simulink model "SOC_model_Code_Gen"  (R2025a)
settings: Solver=FixedStepDiscrete  StartTime=0.0  StopTime=10.0  FixedStep=1  RelTol=1e-3
InitFcn:
  | clear
  | S = load("01_TEST_LGHG2@n10degC_Norm_(05_Inputs).mat");
  | steps = size(S.X,2);
  | t = (0:(steps-1))';
  | X_in = timeseries(single(S.X'), t);
  | true_SOC = timeseries(single(S.Y'), t);
libraries: deeplib x3
settings OptimizationCC: DefaultParameterBehavior=Inlined  EnhancedBackFolding=on  PassReuseOutputArgsAs=Individual arguments  ZeroExternalMemoryAtStartup=off  ZeroInternalMemoryAtStartup=off  OptimizeBlockOrder=speed  DifferentSizesBufferReuse=on  OptimizationCustomize=off  EfficientTunableParamExpr=on
settings DebuggingCC: ParameterTunabilityLossMsg=error
settings HardwareCC: ProdBitPerLong=64.0  ProdHWDeviceType=Intel->x86-64 (Linux 64)
settings SFSimCC: MATLABDynamicMemAlloc=off  SimTargetLang=C++  SimDLTargetLibrary=mkl-dnn
settings RTWCC: SystemTargetFile=ert.tlc  TemplateMakefile=ert_default_tmf  PortableWordSizes=on  CodeProfilingInstrumentation=coarse  Description=Embedded Coder
settings CodeAppCC: ForceParamTrailComments=on  IgnoreCustomStorageClasses=off  OperatorAnnotations=on  SimulinkDataObjDesc=on  SFDataObjDesc=on  InsertBlockDesc=on
settings ERTTargetCC: ExtModeTransport=0.0  ExtModeStaticAlloc=off  ExtModeMexFile=ext_comm  ExtModeIntrfLevel=Level1  ERTCustomFileTemplate=example_file_process.tlc  TargetLangStandard=C99 (ISO)  GenerateSampleERTMain=on  SupportVariableSizeSignals=on

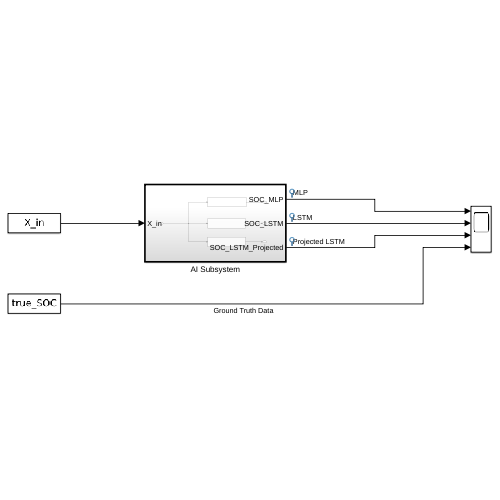
[thumbnail: Simulink's stored preview of the top-level diagram]
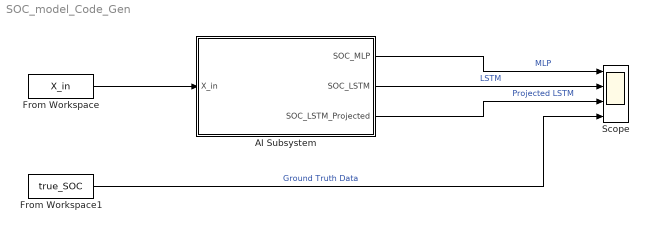
== system SOC_model_Code_Gen ==
  AI Subsystem : Subsystem  TreatAsAtomicUnit=on
      settings: RTWSystemCode=Nonreusable function
  From Workspace : FromWorkspace  VariableName=X_in  SampleTime=1
  From Workspace1 : FromWorkspace  VariableName=true_SOC  SampleTime=1
  Scope : Scope  NumInputPorts=4
      settings: ActiveDisplayYMinimum=0.87097  ActiveDisplayYMaximum=1.01799
  wires:
  AI Subsystem/1(SOC_MLP) -> Scope/1  "MLP"
  AI Subsystem/3(SOC_LSTM_Projected) -> Scope/3  "Projected LSTM"
  AI Subsystem/2(SOC_LSTM) -> Scope/2  "LSTM"
  From Workspace/1 -> AI Subsystem/1(X_in)
  From Workspace1/1 -> Scope/4  "Ground Truth Data"

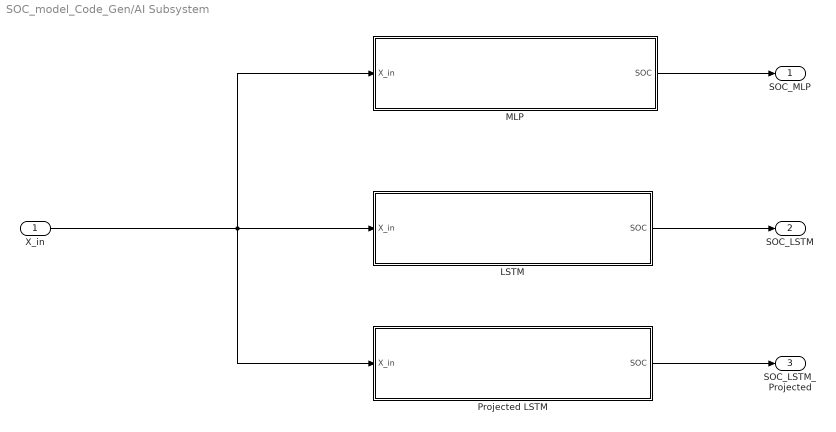
== system SOC_model_Code_Gen/AI Subsystem ==
  X_in : Inport
  LSTM : Subsystem  TreatAsAtomicUnit=on
      settings: RTWSystemCode=Nonreusable function
  MLP : Subsystem  TreatAsAtomicUnit=on
      settings: RTWSystemCode=Nonreusable function
  Projected LSTM : Subsystem  TreatAsAtomicUnit=on
      settings: RTWSystemCode=Nonreusable function
  SOC_MLP : Outport
  SOC_LSTM : Outport  Port=2
  SOC_LSTM_Projected : Outport  Port=3
  wires:
  Projected LSTM/1(SOC) -> SOC_LSTM_Projected/1
  LSTM/1(SOC) -> SOC_LSTM/1
  MLP/1(SOC) -> SOC_MLP/1
  X_in/1 -> MLP/1(X_in), LSTM/1(X_in), Projected LSTM/1(X_in)

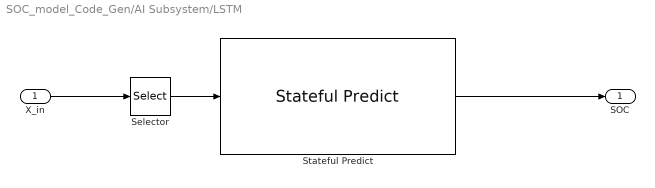
== system SOC_model_Code_Gen/AI Subsystem/LSTM ==
  X_in : Inport
  Selector : Selector  InputPortWidth=5  IndexOptions=Index vector (dialog)  Indices=[1 2 3]  OutputSizes=1
  Stateful Predict : deeplib/Stateful Predict  Network=Network from MAT-file  NetworkFunction=untitled  NetworkFilePath=DLmodel_ref_stackedLSTM.mat  InputDataFormats={ 'sequenceinput', 'CBT' }  SampleTime=-1  ForceInterpretedSim=off  EnableDLNetwork=on  LastKnownNetworkFilePath=''  LastKnownNetworkTimeStamp=''
  SOC : Outport
  wires:
  X_in/1 -> Selector/1
  Stateful Predict/1 -> SOC/1
  Selector/1 -> Stateful Predict/1

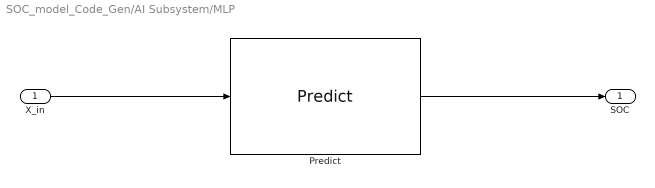
== system SOC_model_Code_Gen/AI Subsystem/MLP ==
  X_in : Inport
  Predict : deeplib/Predict  Network=Network from MAT-file  NetworkFunction=squeezenet  NetworkFilePath=trainedNetwork.mat  MiniBatchSize=128  InputDataFormats={ 'featureinput', 'CB' }  Predictions=on  Activations={}  ForceInterpretedSim=off  EnableDLNetwork=on  LastKnownNetworkFilePath=''  LastKnownNetworkTimeStamp=''
  SOC : Outport
  wires:
  Predict/1 -> SOC/1
  X_in/1 -> Predict/1

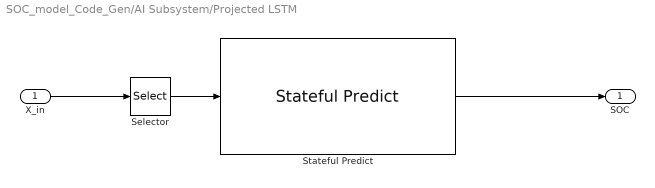
== system SOC_model_Code_Gen/AI Subsystem/Projected LSTM ==
  X_in : Inport
  Selector : Selector  InputPortWidth=5  IndexOptions=Index vector (dialog)  Indices=[1 2 3]  OutputSizes=1
  Stateful Predict : deeplib/Stateful Predict  Network=Network from MAT-file  NetworkFunction=untitled  NetworkFilePath=DLmodel_ref_stackedLSTM_Projected.mat  InputDataFormats={ 'sequenceinput', 'CBT' }  SampleTime=-1  ForceInterpretedSim=off  EnableDLNetwork=on  LastKnownNetworkFilePath=''  LastKnownNetworkTimeStamp=''
  SOC : Outport
  wires:
  Selector/1 -> Stateful Predict/1
  Stateful Predict/1 -> SOC/1
  X_in/1 -> Selector/1
